simulink model "Sim_NL_XZ"  (R2016a)
settings: Solver=VariableStepAuto  StartTime=0.0  StopTime=2  RelTol=1e-3
settings Model: Creator=Florian  LastModifiedBy=Florian

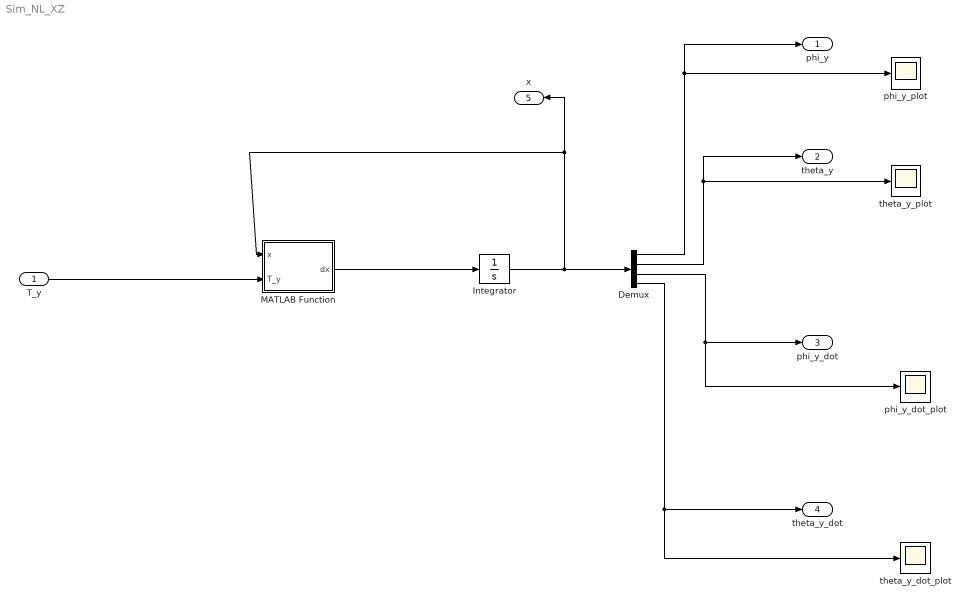
== system Sim_NL_XZ ==
  "T_y " : Inport
  Demux : Demux
  Integrator : Integrator  InitialCondition=[0;0; 0; 0]
  MATLAB Function : MATLAB Function  TreatAsAtomicUnit=on
  phi_y_dot_plot : Scope
  phi_y_plot : Scope
  theta_y_dot_plot : Scope
  theta_y_plot : Scope
  phi_y : Outport
  theta_y : Outport  Port=2
  phi_y_dot : Outport  Port=3
  theta_y_dot : Outport  Port=4
  x : Outport  Port=5
  wires:
  MATLAB Function/1(dx) -> Integrator/1
  Integrator/1 -> x/1, MATLAB Function/1(x), Demux/1
  Demux/1 -> phi_y_plot/1, phi_y/1
  Demux/2 -> theta_y/1, theta_y_plot/1
  Demux/3 -> phi_y_dot_plot/1, phi_y_dot/1
  Demux/4 -> theta_y_dot_plot/1, theta_y_dot/1
  "T_y "/1 -> MATLAB Function/2(T_y)

== matlab function Sim_NL_XZ/MATLAB Function ==
  data: x input; T_y input; dx output
function dx = fcn_xz(x,T_y)

%Zuweisung Koordinaten und Ableitungen
phi_y =x(1);
theta_y=x(2);
phi_y_dot=x(3);
theta_y_dot=x(4);

phi_y_dotdot=(18014398509481984*(1474780203060832382832000000*sin(theta_y)*theta_y_dot^2 + 6673461925215283943359375000*T_y + 295268271287815685091301875*sin(theta_y) - 8944396862587810826384572416*cos(theta_y)*sin(theta_y) + 517041384719804006400000000*T_y*cos(theta_y)))/(75*(1807366736725976544289483038067261440000*cos(theta_y) - 27374775655728371289468879137739903074304*cos(theta_y)^2 + 200948944860727701207841270280447671484375));

theta_y_dotdot= -(9007199254740992*(22102728721212020468750000*T_y - 405980752992200943301368000*sin(theta_y) - 300987024758221901214375*theta_y_dot^2*sin(theta_y) + 41363310777584320512000000*T_y*cos(theta_y) + 9117631868081356601819136*theta_y_dot^2*cos(theta_y)*sin(theta_y)))/(3*(1807366736725976544289483038067261440000*cos(theta_y) - 27374775655728371289468879137739903074304*cos(theta_y)^2 + 200948944860727701207841270280447671484375));

%Zuweisung Ausgang
dx = [phi_y_dot; theta_y_dot; phi_y_dotdot; theta_y_dotdot];
end
